simulink subsystem "Tank"  (R2022a)
settings: Solver=VariableStepAuto  StartTime=0.0  StopTime=10.0  RelTol=1e-3
settings Model: Creator=mmarq  LastModifiedBy=mmarq

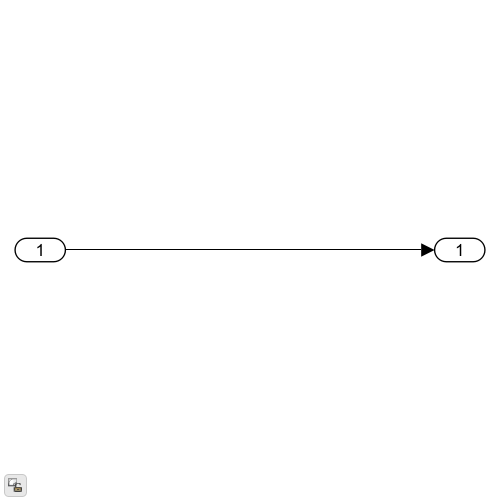
[thumbnail: Simulink's stored preview of the top-level diagram]
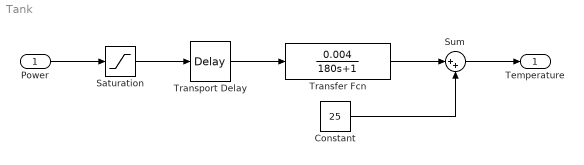
== system Tank ==
  Power : Inport
  Constant : Constant  Value=25
  Saturation : Saturate  UpperLimit=5000  LowerLimit=0
  Sum : Sum  Inputs=|++
  Transfer Fcn : TransferFcn  Numerator=[0.004]  Denominator=[180 1]
  Transport Delay : TransportDelay  DelayTime=5
  Temperature : Outport
  wires:
  Transport Delay/1 -> Transfer Fcn/1
  Constant/1 -> Sum/2
  Power/1 -> Saturation/1
  Saturation/1 -> Transport Delay/1
  Transfer Fcn/1 -> Sum/1
  Sum/1 -> Temperature/1
